simulink model "SML_NonLinear"  (R2018b)
settings: Solver=FixedStepAuto  StartTime=0.0  StopTime=10  FixedStep=0.01  RelTol=1e-3
settings Model: Creator=user  LastModifiedBy=user

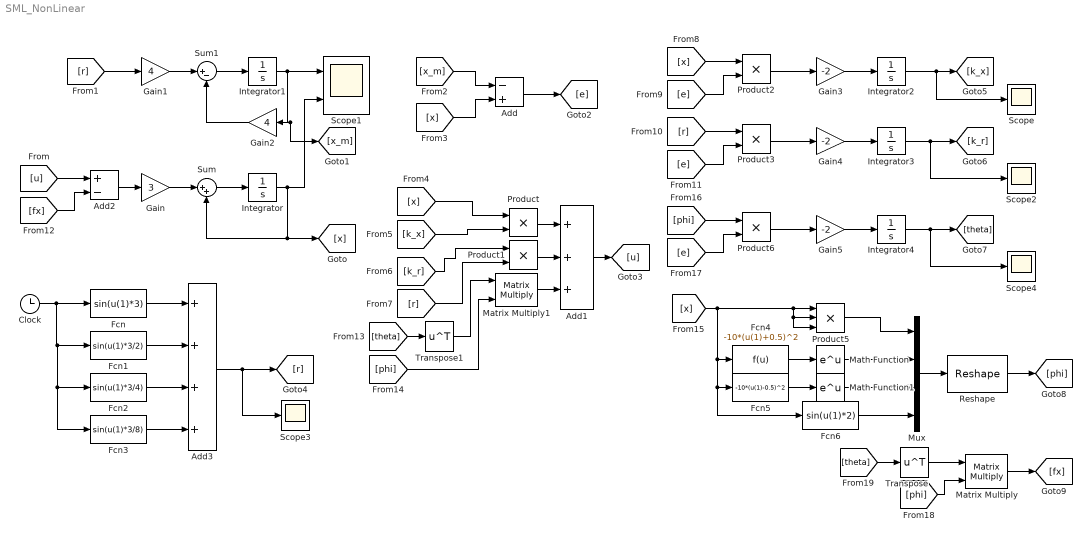
== system SML_NonLinear ==
  Add : Sum  Inputs=-+
  Add1 : Sum  Inputs=+++
  Add2 : Sum  Inputs=+-
  Add3 : Sum  Inputs=++++
  Clock : Clock
  Fcn : Fcn  Expr=sin(u(1)*3)
  Fcn1 : Fcn  Expr=sin(u(1)*3/2)
  Fcn2 : Fcn  Expr=sin(u(1)*3/4)
  Fcn3 : Fcn  Expr=sin(u(1)*3/8)
  Fcn4 : Fcn  Expr=-10*(u(1)+0.5)^2
  Fcn5 : Fcn  Expr=-10*(u(1)-0.5)^2
  Fcn6 : Fcn  Expr=sin(u(1)*2)
  Gain : Gain  Gain=3
  Gain1 : Gain  Gain=4
  Gain2 : Gain  Gain=4
  Gain3 : Gain  Gain=-2
  Gain4 : Gain  Gain=-2
  Gain5 : Gain  Gain=-2
  Integrator{,1..4} (5 alike) : Integrator
  Math Function : Math  SaturateOnIntegerOverflow=on
  Math Function1 : Math  SaturateOnIntegerOverflow=on
  Matrix Multiply : Product  Multiplication=Matrix(*)
  Matrix Multiply1 : Product  Multiplication=Matrix(*)
  Mux : Mux
  Product{,1..3,6} (5 alike) : Product
  Product5 : Product  Inputs=3
  Reshape : Reshape  OutputDimensionality=Customize  OutputDimensions=[4,1]
  Scope{,2..4} (4 alike) : Scope
  Scope1 : Scope  NumInputPorts=2
  Sum : Sum  Inputs=|++
  Sum1 : Sum  Inputs=|+-
  Transpose : Math  Operator=transpose  SaturateOnIntegerOverflow=on
  Transpose1 : Math  Operator=transpose  SaturateOnIntegerOverflow=on
  wires:
  Clock/1 -> Fcn3/1, Fcn2/1, Fcn1/1, Fcn/1
  Gain2/1 -> Sum1/2
  Integrator/1 -> Scope1/2, [x], Sum/2
  Gain/1 -> Sum/1
  Sum1/1 -> Integrator1/1
  Gain1/1 -> Sum1/1
  Add/1 -> [e]
  [x] -> Add/2
  Sum/1 -> Integrator/1
  [x_m] -> Add/1
  [r] -> Gain1/1
  Integrator1/1 -> Gain2/1, [x_m], Scope1/1
  Add2/1 -> Gain/1
  [u] -> Add2/1
  [fx] -> Add2/2
  Fcn/1 -> Add3/1
  Fcn1/1 -> Add3/2
  Fcn2/1 -> Add3/3
  Fcn3/1 -> Add3/4
  Add3/1 -> Scope3/1, [r]
  Add1/1 -> [u]
  Product/1 -> Add1/1
  Product1/1 -> Add1/2
  Matrix Multiply1/1 -> Add1/3
  [x] -> Product/1
  [k_x] -> Product/2
  [k_r] -> Product1/1
  [r] -> Product1/2
  [x] -> Product2/1
  [e] -> Product2/2
  Product2/1 -> Gain3/1
  Gain3/1 -> Integrator2/1
  Integrator2/1 -> Scope/1, [k_x]
  [r] -> Product3/1
  [e] -> Product3/2
  Product3/1 -> Gain4/1
  Gain4/1 -> Integrator3/1
  Integrator3/1 -> Scope2/1, [k_r]
  [x] -> Fcn6/1, Fcn5/1, Fcn4/1, Product5/2, Product5/3, Product5/1
  Product5/1 -> Mux/1
  Mux/1 -> Reshape/1
  Math Function/1 -> Mux/2
  Fcn4/1 -> Math Function/1
  Fcn5/1 -> Math Function1/1
  Math Function1/1 -> Mux/3
  Fcn6/1 -> Mux/4
  Reshape/1 -> [phi]
  Product6/1 -> Gain5/1
  [e] -> Product6/2
  [phi] -> Product6/1
  Integrator4/1 -> Scope4/1, [theta]
  Gain5/1 -> Integrator4/1
  Matrix Multiply/1 -> [fx]
  [theta] -> Transpose/1
  Transpose/1 -> Matrix Multiply/1
  [phi] -> Matrix Multiply/2
  [theta] -> Transpose1/1
  [phi] -> Matrix Multiply1/2
  Transpose1/1 -> Matrix Multiply1/1
